simulink model "mixreceiver"  (R2013a)
settings: Solver=ode45  StartTime=0.0  StopTime=10.0  RelTol=1e-3
libraries: commcrc2 x2, commrandsrc2 x1
settings Model: Creator=chenhr  LastModifiedBy=chenhr

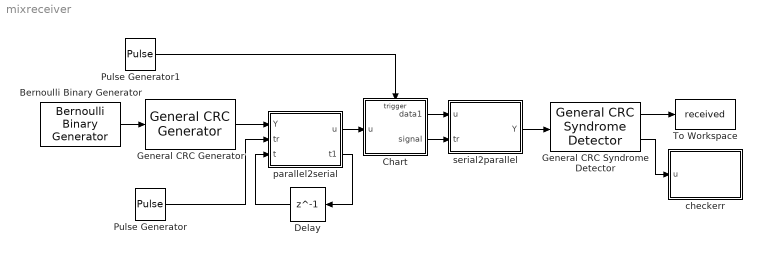
== system mixreceiver ==
  Bernoulli Binary Generator : commrandsrc2/Bernoulli Binary Generator  P=0.5  seed=61  Ts=1  frameBased=on  sampPerFrame=64  orient=off  outDataType=double
  Chart : Stateflow chart  TreatAsAtomicUnit=on
  Delay : Delay  DelayLength=1
  General CRC Generator : commcrc2/General CRC Generator  genPoly=[1 0 0 0 1 0 0 0 0 0 0 1 0 0 0 0 1]  iniStates=0  directMethod=off  reflectInputBytes=off  reflectChecksums=off  finalXOR=0  numChecksums=1
  General CRC Syndrome Detector : commcrc2/General CRC Syndrome Detector  genPoly=[1 0 0 0 1 0 0 0 0 0 0 1 0 0 0 0 1]  iniStates=0  directMethod=off  reflectInputBytes=off  reflectChecksums=off  finalXOR=0  numChecksums=1
  Pulse Generator : DiscretePulseGenerator  Period=300  PhaseDelay=10  SampleTime=0.01
  Pulse Generator1 : DiscretePulseGenerator  SampleTime=0.005
  To Workspace : ToWorkspace  VariableName=received  SampleTime=-1  SaveFormat=Timeseries
  checkerr : MATLAB Function  TreatAsAtomicUnit=on
  parallel2serial : MATLAB Function  TreatAsAtomicUnit=on  SystemSampleTime=0.01
  serial2parallel : MATLAB Function  TreatAsAtomicUnit=on  SystemSampleTime=0.01
  wires:
  Bernoulli Binary Generator/1 -> General CRC Generator/1
  parallel2serial/2(t1) -> Delay/1
  Delay/1 -> parallel2serial/3(t)
  General CRC Generator/1 -> parallel2serial/1(Y)
  Pulse Generator/1 -> parallel2serial/2(tr)
  parallel2serial/1(u) -> Chart/1(u)
  Chart/1(data1) -> serial2parallel/1(u)
  serial2parallel/1(Y) -> General CRC Syndrome Detector/1
  Chart/2(signal) -> serial2parallel/2(tr)
  Pulse Generator1/1 -> Chart/Trigger
  General CRC Syndrome Detector/1 -> To Workspace/1
  General CRC Syndrome Detector/2 -> checkerr/1(u)

== stateflow chart mixreceiver/Chart ==
  state x4
  state z5
  state z6
  state x3
  state z7
  state z8
  state z9
  state x1
  state x2
  state z10
  state z11
  state z12
  state z13
  state wait
    en:
    signal=0;
  state z14
  state z16
  state z15
  state g
    en:
    signal = 1;
  state z17
  state error
  state receive
  state e
  state b
    ex:
    data1=0;
  state a
  state d
    ex:
    data1=1;
  state f
  state c
  x4 -> z5 [order 2] : [u==0]
  x3 -> x4 [order 1] : [u==1]
  x4 -> wait [order 1] : [u==1]
  z5 -> z6 : [u==0]
  (default) -> x3 [order 2] : [u==1]
  z6 -> z7 [order 1] : [u==0]
  (default) -> wait [order 1]
  z9 -> z10 [order 2] : [u==1]
  z6 -> wait [order 2] : [u==1]
  z7 -> z8 [order 2] : [u==1]
  x3 -> x2 [order 2] : [u==0]
  z8 -> z9 [order 2] : [u==1]
  x2 -> x3 [order 2] : [u==1]
  z11 -> x3 [order 1] : [u==1]
  z7 -> wait [order 1] : [u==0]
  z9 -> x2 [order 1] : [u==0]
  z8 -> x2 [order 1] : [u==0]
  z10 -> z11 [order 2] : [u==0]
  x1 -> x2 [order 1] : [u==0]
  z10 -> wait [order 1] : [u==1]
  x1 -> x1 [order 2] : [u==1]
  wait -> x1 [order 1] : [u==1]
  x2 -> wait [order 1] : [u==0]
  z11 -> z12 [order 2] : [u==0]
  z12 -> wait [order 1] : [u==1]
  z12 -> z13 [order 2] : [u==0]
  wait -> wait [order 2] : [u==0]
  z13 -> wait [order 1] : [u==0]
  z13 -> z14 [order 2] : [u==1]
  z15 -> wait [order 2] : [u==0]
  z17 -> wait [order 1] : [u==0]
  z16 -> wait [order 1] : [u==1]
  z14 -> wait [order 1] : [u==1]
  error -> wait
  g -> wait
  z14 -> z15 [order 2] : [u==0]
  z15 -> z16 [order 1] : [u==1]
  z16 -> z17 [order 2] : [u==0]
  z17 -> receive [order 2] : [u==1]
  f -> g [order 1] : [u==1]
  e -> error [order 2] : [u==0]
  c -> error [order 2] : [u==1]
  f -> error [order 2] : [u==0]
  a -> e [order 2] : [u==0]
  receive -> a [order 1] : [u==0]
  receive -> c [order 2] : [u==1]
  a -> b [order 1] : [u==1]
  b -> a [order 1] : [u==0]
  e -> f [order 1] : [u==1]
  d -> a [order 2] : [u==0]
  b -> c [order 2] : [u==1]
  c -> d [order 1] : [u==0]
  d -> c [order 1] : [u==1]
  data: data1 output double; u input; signal output double
  events: event input RISING_EDGE_EVENT

== matlab function mixreceiver/parallel2serial ==
  data: u output; Y input; tr input; t input; t1 output
function [u, t1]  = fcn(Y, tr, t)
N = 80;
persistent q;
if isempty(q)
    q = zeros(N * 2 + 22, 1);
end
if tr == 0
    if t < N * 2 + 22
        t = t + 1;
        u = q(t);
        t1 = t;
    else 
        u = 0;
        t1 = t;
    end
else
    q(1:18, 1) = [1, 0, 1, 1, 0, 0, 0, 1, 1, 1, 0, 0, 0, 1, 0, 1, 0, 1]';
    for i = 1:N
        if Y(i) == 0
            q(17 + i * 2) = 0;
            q(18 + i * 2) = 1;
        else
            q(17 + i * 2) = 1;
            q(18 + i * 2) = 0;
        end
    end
    q((19 + 2 * N):(22 + 2 * N), 1) = [0, 0, 1, 1]';
    t = 1;
    u = q(t);
    t1 = t;
end

== matlab function mixreceiver/serial2parallel ==
  data: u input; Y output; tr input
function Y  = fcn(u, tr)
N = 81;
persistent q;
if isempty(q)
    q = zeros(N * 2, 1);
end
if tr == 0
    for t = 1:(N * 2 -1)
        q(t) = q(t+1);
    end
    q(N * 2) = u;
    Y = zeros(N - 1, 1);
else
    Y = zeros(N - 1, 1);
    for t = 1:(N - 1)
        Y(t) = q(t * 2);
    end
end

== matlab function mixreceiver/checkerr ==
  data: u input
function fcn(u)
if u ~= 0
    fprintf('CRC Verification Failed!\n');
end
